simulink model "backbone"  (R2022b)
settings: Solver=FixedStepDiscrete  StartTime=0.0  StopTime=2  FixedStep=0.000001  RelTol=1e-3
undefined symbols (not defined in the file or in its folder): DiscIntNeverNeededParam, flux, Motor_flux, Motor_Ld_Indctances, Motor_Lq_Indctances, Motor_Pn, Motor_Rs, Pn, switch_electronic_feedworward, Switch_SubsysCtrl, SysCurrentMax, SysVoltage, Ts
libraries: powerlib_extras x11, simulink x4, mcbcontrolslib x4, slpidlib x3, spsPermanentMagnetSynchronousMachineLib x2, spsDCVoltageSourceLib x2, spsGroundLib x1, eePmsmCurrentController x1, spsThreePhaseVIMeasurementLib x1, spsTwoLevelConverterLib x1, spsUniversalBridgeLib x1, spspowerguiLib x1
(part 2 of 3)

== system backbone/Variant Subsystem/DTC_PMSM/PWM ==
  N : Inport
  Flux : Inport  Port=2
  Torque : Inport  Port=3
  Data Type Conversion : DataTypeConversion  OutDataTypeStr=boolean  SaturateOnIntegerOverflow=off  RndMeth=Floor
  Data Type Conversion1 : DataTypeConversion  OutDataTypeStr=boolean  SaturateOnIntegerOverflow=off  RndMeth=Floor
  Data Type Conversion2 : DataTypeConversion  OutDataTypeStr=boolean  SaturateOnIntegerOverflow=off  RndMeth=Floor
  Logical Operator3 : Logic  Operator=NOT  AllPortsSameDT=off  OutDataTypeStr=boolean
  Logical Operator4 : Logic  Operator=NOT  AllPortsSameDT=off  OutDataTypeStr=boolean
  Logical Operator5 : Logic  Operator=NOT  AllPortsSameDT=off  OutDataTypeStr=boolean
  Lookup Table : Lookup  InputValues=[1,2,3,4,5,6]  Table=[1,1,0,0,0,1]  SaturateOnIntegerOverflow=off
  Lookup Table1 : Lookup  InputValues=[1,2,3,4,5,6]  Table=[0,1,1,1,0,0]  SaturateOnIntegerOverflow=off
  Lookup Table2 : Lookup  InputValues=[1,2,3,4,5,6]  Table=[0,0,0,1,1,1]  SaturateOnIntegerOverflow=off
  Mux1 : Mux  Inputs=6
  PMSM_switch : MATLAB Function  TreatAsAtomicUnit=on
  pluse : Outport
  wires:
  Logical Operator3/1 -> Mux1/2
  Logical Operator4/1 -> Mux1/4
  Logical Operator5/1 -> Mux1/6
  Mux1/1 -> pluse/1
  PMSM_switch/1(Table) -> Lookup Table1/1, Lookup Table/1, Lookup Table2/1
  Lookup Table/1 -> Data Type Conversion/1
  Data Type Conversion/1 -> Mux1/1, Logical Operator3/1
  Lookup Table1/1 -> Data Type Conversion1/1
  Data Type Conversion1/1 -> Mux1/3, Logical Operator4/1
  Lookup Table2/1 -> Data Type Conversion2/1
  Data Type Conversion2/1 -> Mux1/5, Logical Operator5/1
  Flux/1 -> PMSM_switch/1(Flux)
  Torque/1 -> PMSM_switch/2(Torque)
  N/1 -> PMSM_switch/3(N)

== system backbone/Variant Subsystem/DTC_PMSM/Speed2 ==
  note: Pierre Giroux, Gilbert Sybille
      | Power System Simulation Laboratory
      | IREQ, Hydro-Quebc
  note: Discrete PID Controller
  Error : Inport  SampleTime=Ts
  Discrete-Time Integrator : DiscreteIntegrator  InitialCondition=Init  SampleTime=Ts  LimitOutput=on  UpperSaturationLimit=UpperLimit  LowerSaturationLimit=LowerLimit  ICPrevOutput=DiscIntNeverNeededParam  ICPrevScaledInput=DiscIntNeverNeededParam
  Kp1 : Gain  Gain=Ba  SaturateOnIntegerOverflow=on  SampleTime=Ts  OutDataTypeStr=Inherit: Same as input  ParamDataTypeStr=Inherit: Same as input
  Kp4 : Gain  Gain=Kpw  SaturateOnIntegerOverflow=on  SampleTime=Ts  OutDataTypeStr=Inherit: Same as input  ParamDataTypeStr=Inherit: Same as input
  Kp5 : Gain  Gain=Kiw  SaturateOnIntegerOverflow=on  SampleTime=Ts  OutDataTypeStr=Inherit: Same as input  ParamDataTypeStr=Inherit: Same as input
  Saturation2 : Saturate  UpperLimit=UpperLimit  LowerLimit=LowerLimit  SampleTime=Ts
  Sum6 : Sum  Inputs=++-  InputSameDT=on  SaturateOnIntegerOverflow=on  SampleTime=Ts  OutDataTypeStr=Inherit: Same as first input
  Zero-Order Hold : ZeroOrderHold  SampleTime=Ts
  Out : Outport  SampleTime=Ts  InitialOutput=0
  wires:
  Kp1/1 -> Sum6/3
  Sum6/1 -> Saturation2/1
  Kp5/1 -> Discrete-Time Integrator/1
  Kp4/1 -> Zero-Order Hold/1
  Discrete-Time Integrator/1 -> Sum6/2
  Saturation2/1 -> Out/1
  Zero-Order Hold/1 -> Sum6/1
  Error/1 -> Kp4/1, Kp5/1, Kp1/1

== system backbone/Variant Subsystem/DTC_PMSM/定子磁链和电磁转矩估计 ==
  note: 1) Add Subsystem or Model blocks as valid variant choices.
      | 2) You cannot connect blocks at this level. At simulation, connectivity is automatically
      | determined, based on the active variant and port name matching.
  Iα : Inport
  iβ : Inport  Port=2
  扩展卡尔曼滤波磁链估计 : Subsystem  VariantControl=DTC_Flux_Predict==2
  电压法估计磁链 : Subsystem  VariantControl=DTC_Flux_Predict==0
  N : Outport
  φ_est : Outport  Port=2
  Te_est : Outport  Port=3

== system backbone/Variant Subsystem/DTC_SVPWM_PMSM/速度pi1 ==
  note: Discrete PID Controller
  note: Pierre Giroux, Gilbert Sybille
      | Power System Simulation Laboratory
      | IREQ, Hydro-Quebc
  Error : Inport  SampleTime=Ts
  Discrete-Time Integrator : DiscreteIntegrator  InitialCondition=Init  SampleTime=Ts  LimitOutput=on  UpperSaturationLimit=UpperLimit  LowerSaturationLimit=LowerLimit  ICPrevOutput=DiscIntNeverNeededParam  ICPrevScaledInput=DiscIntNeverNeededParam
  Kp1 : Gain  Gain=Ba  SaturateOnIntegerOverflow=on  SampleTime=Ts  OutDataTypeStr=Inherit: Same as input  ParamDataTypeStr=Inherit: Same as input
  Kp4 : Gain  Gain=Kpw  SaturateOnIntegerOverflow=on  SampleTime=Ts  OutDataTypeStr=Inherit: Same as input  ParamDataTypeStr=Inherit: Same as input
  Kp5 : Gain  Gain=Kiw  SaturateOnIntegerOverflow=on  SampleTime=Ts  OutDataTypeStr=Inherit: Same as input  ParamDataTypeStr=Inherit: Same as input
  Saturation2 : Saturate  UpperLimit=UpperLimit  LowerLimit=LowerLimit  SampleTime=Ts
  Sum6 : Sum  Inputs=++-  InputSameDT=on  SaturateOnIntegerOverflow=on  SampleTime=Ts  OutDataTypeStr=Inherit: Same as first input
  Zero-Order Hold : ZeroOrderHold  SampleTime=Ts
  Out : Outport  SampleTime=Ts  InitialOutput=0
  wires:
  Error/1 -> Kp1/1, Kp5/1, Kp4/1
  Zero-Order Hold/1 -> Sum6/1
  Saturation2/1 -> Out/1
  Discrete-Time Integrator/1 -> Sum6/2
  Kp4/1 -> Zero-Order Hold/1
  Kp5/1 -> Discrete-Time Integrator/1
  Sum6/1 -> Saturation2/1
  Kp1/1 -> Sum6/3

== system backbone/Variant Subsystem/DTC_SVPWM_PMSM/速度pi2 ==
  note: Pierre Giroux, Gilbert Sybille
      | Power System Simulation Laboratory
      | IREQ, Hydro-Quebc
  note: Discrete PID Controller
  Error : Inport  SampleTime=Ts
  Discrete-Time Integrator : DiscreteIntegrator  InitialCondition=Init  SampleTime=Ts  LimitOutput=on  UpperSaturationLimit=UpperLimit  LowerSaturationLimit=LowerLimit  ICPrevOutput=DiscIntNeverNeededParam  ICPrevScaledInput=DiscIntNeverNeededParam
  Kp1 : Gain  Gain=Ba  SaturateOnIntegerOverflow=on  SampleTime=Ts  OutDataTypeStr=Inherit: Same as input  ParamDataTypeStr=Inherit: Same as input
  Kp4 : Gain  Gain=Kpw  SaturateOnIntegerOverflow=on  SampleTime=Ts  OutDataTypeStr=Inherit: Same as input  ParamDataTypeStr=Inherit: Same as input
  Kp5 : Gain  Gain=Kiw  SaturateOnIntegerOverflow=on  SampleTime=Ts  OutDataTypeStr=Inherit: Same as input  ParamDataTypeStr=Inherit: Same as input
  Saturation2 : Saturate  UpperLimit=UpperLimit  LowerLimit=LowerLimit  SampleTime=Ts
  Sum6 : Sum  Inputs=++-  InputSameDT=on  SaturateOnIntegerOverflow=on  SampleTime=Ts  OutDataTypeStr=Inherit: Same as first input
  Zero-Order Hold : ZeroOrderHold  SampleTime=Ts
  Out : Outport  SampleTime=Ts  InitialOutput=0
  wires:
  Kp1/1 -> Sum6/3
  Sum6/1 -> Saturation2/1
  Kp5/1 -> Discrete-Time Integrator/1
  Kp4/1 -> Zero-Order Hold/1
  Discrete-Time Integrator/1 -> Sum6/2
  Saturation2/1 -> Out/1
  Zero-Order Hold/1 -> Sum6/1
  Error/1 -> Kp4/1, Kp5/1, Kp1/1

== system backbone/Variant Subsystem/MPTA_MPTV_PMSM/Back Electromotive Force ==
  note: (We*Lq*iq)
  note: We*flux
  note: (We*Ld*id)
  we : Inport
  iq : Inport  Port=2
  id : Inport  Port=3
  Constant : Constant  Value=0
  Constant1 : Constant  Value=switch_electronic_feedworward
  Gain : Gain  Gain=Motor_Ld_Indctances
  Gain1 : Gain  Gain=Motor_flux
  Gain2 : Gain  Gain=Motor_Lq_Indctances
  Product : Product
  Product1 : Product
  Sum : Sum
  Switch : Switch  Criteria=u2 > Threshold  SaturateOnIntegerOverflow=off  InputSameDT=off
  E_d : Outport
  E_q : Outport  Port=2
  wires:
  Switch/1 -> Gain1/1, Gain/1, Gain2/1
  Product1/1 -> E_d/1
  Gain1/1 -> Sum/1
  Sum/1 -> E_q/1
  Product/1 -> Sum/2
  Constant1/1 -> Switch/2
  id/1 -> Product/2
  iq/1 -> Product1/2
  Gain2/1 -> Product1/1
  Gain/1 -> Product/1
  we/1 -> Switch/1
  Constant/1 -> Switch/3

== system backbone/Variant Subsystem/MPTA_MPTV_PMSM/MPTA_弱磁 ==
  note: 1) Add Subsystem or Model blocks as valid variant choices.
      | 2) You cannot connect blocks at this level. At simulation, connectivity is automatically
      | determined, based on the active variant and port name matching.
  input : Inport
  "MPTA_MPTV_Base_IMax " : Subsystem  VariantControl=true
  MPTA_MPTV_Base_Te : Subsystem  VariantControl=false
  id_ref : Outport
  iq_ref : Outport  Port=2

== system backbone/Variant Subsystem/SMC_OR_PID/Back Electromotive Force ==
  note: (We*Ld*id)
  note: (We*flux)
  note: (We*Lq*iq)
  we : Inport
  iq : Inport  Port=2
  id : Inport  Port=3
  Constant : Constant  Value=0
  Constant1 : Constant  Value=switch_electronic_feedworward
  Gain : Gain  Gain=Motor_Ld_Indctances
  Gain1 : Gain  Gain=Motor_flux
  Gain2 : Gain  Gain=Motor_Lq_Indctances
  Product : Product
  Product1 : Product
  Sum : Sum
  Switch : Switch  Criteria=u2 > Threshold  SaturateOnIntegerOverflow=off  InputSameDT=off
  E_d : Outport
  E_q : Outport  Port=2
  wires:
  Gain/1 -> Product/1
  Gain2/1 -> Product1/1
  iq/1 -> Product1/2
  id/1 -> Product/2
  Constant1/1 -> Switch/2
  Product/1 -> Sum/2
  Sum/1 -> E_q/1
  Gain1/1 -> Sum/1
  Product1/1 -> E_d/1
  Switch/1 -> Gain2/1, Gain/1, Gain1/1
  Constant/1 -> Switch/3
  we/1 -> Switch/1

== system backbone/Variant Subsystem/SMC_OR_PID/Variant Subsystem ==
  note: 1) Add Subsystem or Model blocks as valid variant choices.
      | 2) You cannot connect blocks at this level. At simulation, connectivity is automatically
      | determined, based on the active variant and port name matching.
  In1 : Inport
  PID : Subsystem  VariantControl=true
  SMC : Subsystem  VariantControl=false
  Te* : Outport

== system backbone/Variant Subsystem/SMC_OR_PID/Variant Subsystem1 ==
  note: 1) Add Subsystem or Model blocks as valid variant choices.
      | 2) You cannot connect blocks at this level. At simulation, connectivity is automatically
      | determined, based on the active variant and port name matching.
  we : Inport
  Te* : Inport  Port=2
  LD=LQ/id=0 : Subsystem  VariantControl=MPTA_SubSysCtrl==0
  MPTA_Process : Subsystem  VariantControl=MPTA_SubSysCtrl==1
  id_ref : Outport
  iq_ref : Outport  Port=2

== system backbone/Variant Subsystem/SMC_OR_PID/Variant Subsystem2 ==
  note: 1) Add Subsystem or Model blocks as valid variant choices.
      | 2) You cannot connect blocks at this level. At simulation, connectivity is automatically
      | determined, based on the active variant and port name matching.
  ialpha : Inport
  ibeta : Inport  Port=2
  ualpha : Inport  Port=3
  ubeta : Inport  Port=4
  Ts : Inport  Port=5
  Ls : Inport  Port=6
  Rs : Inport  Port=7
  flux : Inport  Port=8
  EKF_dq : Subsystem  VariantControl=(Motor_Observer==2)&&(Motor_Ld_Indctances==Motor_Lq_Indctances)
  EKF_αβ : Subsystem  VariantControl=Motor_Observer==0
  Luenberger : Subsystem  VariantControl=Motor_Observer==1
  Model : ModelReference  VariantControl=Choice
  SMO : Subsystem  VariantControl=Motor_Observer==3
  theta : Outport
  we : Outport  Port=2

== system backbone/输出模拟子系统/磁链模拟/Variant Subsystem ==
  note: 1) Add Subsystem or Model blocks as valid variant choices.
      | 2) You cannot connect blocks at this level. At simulation, connectivity is automatically
      | determined, based on the active variant and port name matching.
  In1 : Inport
  Subsystem : Subsystem  VariantControl=true
  Subsystem1 : Subsystem  VariantControl=false
  Out1 : Outport

== system backbone/输出模拟子系统/磁链模拟/clark变换 ==
  note: 基于KCL定律消除Ic 减少一路电流检测，简化clark变换计算过程
  i_a : Inport
  i_b : Inport  Port=2
  i_c : Inport  Port=3
  " 1" : Fcn  Expr=u(1)*(3/2)
  " 1" : Fcn  Expr=u(1)*(sqrt(3)/2)+u(2)*(sqrt(3))
  Mux7 : Mux  Inputs=3
  Alpha : Outport
  Beta : Outport  Port=2
  wires:
  " 1"/1 -> Alpha/1
  " 1"/1 -> Beta/1
  Mux7/1 -> " 1"/1, " 1"/1
  i_a/1 -> Mux7/1
  i_b/1 -> Mux7/2
  i_c/1 -> Mux7/3

== system backbone/输出模拟子系统/磁链模拟/park变换 ==
  Alpha : Inport
  Beta : Inport  Port=2
  We : Inport  Port=3
  " 1" : Fcn  Expr=u(1)*cos(u(3))+u(2)*sin(u(3))
  " 1" : Scope  NumInputPorts=2
  " 1" : Fcn  Expr=-u(1)*sin(u(3))+u(2)*cos(u(3))
  Mux8 : Mux  Inputs=3
  D : Outport
  Q : Outport  Port=2
  wires:
  Alpha/1 -> Mux8/1
  Beta/1 -> Mux8/2
  Mux8/1 -> " 1"/1, " 1"/1
  We/1 -> Mux8/3
  " 1"/1 -> " 1"/1, D/1
  " 1"/1 -> " 1"/2, Q/1

== system backbone/Variant Subsystem/DTC_PMSM/定子磁链和电磁转矩估计/扩展卡尔曼滤波磁链估计 ==
  Iα : Inport
  iβ : Inport  Port=2
  φ_est : Outport
  Te_est : Outport  Port=2
  N : Outport  Port=3

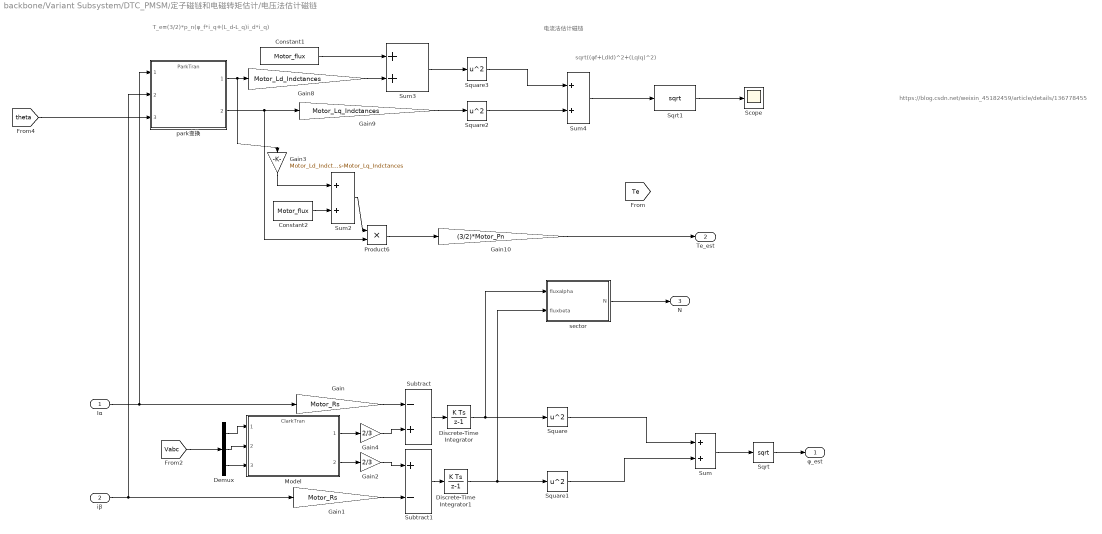
== system backbone/Variant Subsystem/DTC_PMSM/定子磁链和电磁转矩估计/电压法估计磁链 ==
  note: T_e=(3/2)*p_n(φ_f*i_q+(L_d-L_q)i_d*i_q)
  note: 电流法估计磁链
  note: sqrt((φf+LdId)^2+(LqIq)^2)
  note: https://blog.csdn.net/weixin_45182459/article/details/136778455
  Iα : Inport
  iβ : Inport  Port=2
  Constant1 : Constant  Value=Motor_flux
  Constant2 : Constant  Value=Motor_flux
  Demux : Demux  Outputs=3
  Discrete-Time Integrator : DiscreteIntegrator  SampleTime=-1  ICPrevOutput=DiscIntNeverNeededParam  ICPrevScaledInput=DiscIntNeverNeededParam
  Discrete-Time Integrator1 : DiscreteIntegrator  SampleTime=-1  ICPrevOutput=DiscIntNeverNeededParam  ICPrevScaledInput=DiscIntNeverNeededParam
  Gain : Gain  Gain=Motor_Rs
  Gain1 : Gain  Gain=Motor_Rs
  Gain10 : Gain  Gain=(3/2)*Motor_Pn
  Gain2 : Gain  Gain=2/3
  Gain3 : Gain  Gain=Motor_Ld_Indctances-Motor_Lq_Indctances
  Gain4 : Gain  Gain=2/3
  Gain8 : Gain  Gain=Motor_Ld_Indctances
  Gain9 : Gain  Gain=Motor_Lq_Indctances
  Model : ModelReference  ModelNameDialog=ClarkTran.slx  SimulationMode=Normal  ModelReferenceVersion=1.13
  Product6 : Product
  Scope : Scope
  Sqrt : Sqrt
  Sqrt1 : Sqrt
  Square{,1..3} (4 alike) : Math  Operator=square
  Subtract : Sum  Inputs=-+
  Subtract1 : Sum  Inputs=+-
  Sum{,2..4} (4 alike) : Sum
  park变换 : ModelReference  ModelNameDialog=ParkTran.slx  SimulationMode=Normal  ModelReferenceVersion=1.9
  sector : MATLAB Function  TreatAsAtomicUnit=on
  φ_est : Outport
  Te_est : Outport  Port=2
  N : Outport  Port=3
  wires:
  [Vabc] -> Demux/1
  Demux/1 -> Model/1
  Demux/2 -> Model/2
  Demux/3 -> Model/3
  Gain/1 -> Subtract/1
  Gain1/1 -> Subtract1/2
  Subtract/1 -> Discrete-Time Integrator/1
  Subtract1/1 -> Discrete-Time Integrator1/1
  Square/1 -> Sum/1
  Square1/1 -> Sum/2
  Sum/1 -> Sqrt/1
  Sqrt/1 -> φ_est/1
  sector/1(N) -> N/1
  Gain2/1 -> Subtract1/1
  Model/2 -> Gain2/1
  Gain4/1 -> Subtract/2
  Model/1 -> Gain4/1
  Iα/1 -> park变换/1, Gain/1
  Discrete-Time Integrator/1 -> sector/1(fluxalpha), Square/1
  Discrete-Time Integrator1/1 -> sector/2(fluxbeta), Square1/1
  Constant2/1 -> Sum2/2
  park变换/2 -> Product6/2, Gain9/1
  park变换/1 -> Gain3/1, Gain8/1
  Gain8/1 -> Sum3/2
  Constant1/1 -> Sum3/1
  Product6/1 -> Gain10/1
  Sum2/1 -> Product6/1
  Gain3/1 -> Sum2/1
  Square3/1 -> Sum4/1
  Gain9/1 -> Square2/1
  Square2/1 -> Sum4/2
  Sum3/1 -> Square3/1
  Sum4/1 -> Sqrt1/1
  [theta] -> park变换/3
  Sqrt1/1 -> Scope/1
  iβ/1 -> park变换/2, Gain1/1
  Gain10/1 -> Te_est/1

== system backbone/Variant Subsystem/MPTA_MPTV_PMSM/MPTA_弱磁/MPTA_MPTV_Base_IMax  ==
  note: [57.6177 -57.6177]
  note: [50*sqrt(2) -50*sqrt(2)]
  note: https://blog.csdn.net/weixin_44312889/article/details/124467496
  note: https://blog.csdn.net/weixin_44312889/article/details/124467496?ops_request_misc=%257B%2522request%255Fid%2522%253A%2522171975641716800215087501%2522%252C%2522scm%2522%253A%252220140713.130102334.pc%255Fblog.%2522%257D&request_id=171975641716800215087501&biz_id=0&utm_medium=distribute.pc_search_result.none-task-blog-2~blog~first_rank_ecpm_v1~rank_v31_ecpm-23-124467496-null-null.nonecase&utm_term=%20%E5%BC%B1%E7%A3%81%E6%8E%A7%E5%88%B6&spm=1018.2226.3001.4450
  note: https://www.bilibili.com/video/BV1iZ421v75g/?spm_id_from=333.337.search-card.all.click&vd_source=a44fa1878c4911e289ac9693c05baa9b
  note: 此处PID 对应着转速与iq的关系
  input : Inport
  Clock : Clock
  Delay : Delay  DelayLength=1
  LdLqPnFluxRs : Constant  Value=[Motor_Ld_Indctances Motor_Lq_Indctances Motor_Pn Motor_flux Motor_Rs]
  MPTA_MPTV_Imax : MATLAB Function  TreatAsAtomicUnit=on
  MPTA_MPTV_Imax1 : MATLAB Function  Commented=on  TreatAsAtomicUnit=on
  Scope : Scope
  Speed : Subsystem  AncestorBlock=|  DialogController=POWERSYS.PowerSysDialog  mask(Discrete PI Controller){Kpw=0.075, Kiw=0.4, Ba=0, Par_Limits=[57.7 -5], Init=0, Ts=1e-3}
      | powerlib_extras/Discrete 
      | Control Blocks/Discrete
      | PI Controller
      mask prompts: Kpw "Proportional gain (Kp):"; Kiw "Integral gain (Ki):"; Ba "feedback gain (Ba)"; Par_Limits "Output limits: [ Upper   Lower ]"; Init "Output initial value:"; Ts "Sample time:"
      mask help: This block implements a discrete PI controller.
      mask init:
      | UpperLimit=Par_Limits(1);
      | LowerLimit=Par_Limits(2);
      | power_initmask();
      settings: LibrarySourceBlock=|
      | powerlib_extras/Discrete
      | Control Blocks/Discrete
      | PI Controller
      mask Help: This block is part of a subset of blocks in the Extras library that does not have documentation associated with it, other than the block mask description.
      mask Display: disp('PI');
  UI : Constant  Value=[SysVoltage SysCurrentMax]
  iq_ref : Outport
  id_ref : Outport  Port=2
  wires:
  UI/1 -> MPTA_MPTV_Imax/2(UI)
  Delay/1 -> MPTA_MPTV_Imax/6(last_state)
  [we] -> MPTA_MPTV_Imax/5(we)
  Clock/1 -> MPTA_MPTV_Imax/4(clock)
  MPTA_MPTV_Imax/3(state) -> Delay/1
  LdLqPnFluxRs/1 -> MPTA_MPTV_Imax/3(LdLqPnFluxRs)
  input/1 -> Speed/1(Error)
  Speed/1(Out) -> MPTA_MPTV_Imax/1(iqPIDref)
  MPTA_MPTV_Imax/6(Zone) -> Scope/1
  MPTA_MPTV_Imax/2(iqref) -> iq_ref/1
  MPTA_MPTV_Imax/1(idref) -> id_ref/1

== system backbone/Variant Subsystem/MPTA_MPTV_PMSM/MPTA_弱磁/MPTA_MPTV_Base_Te ==
  note: https://blog.csdn.net/qq_54203407/article/details/133353778
  note: https://blog.csdn.net/qq_54203407/article/details/133353778?ops_request_misc=%257B%2522request%255Fid%2522%253A%2522171984152416800225547611%2522%252C%2522scm%2522%253A%252220140713.130102334..%2522%257D&request_id=171984152416800225547611&biz_id=0&utm_medium=distribute.pc_search_result.none-task-blog-2~blog~sobaiduend~default-2-133353778-null-null.nonecase&utm_term=mpta&spm=1018.2226.3001.4450
  note: 此处PID 对应着转速和转矩的关系
  input : Inport
  LdLqPnFluxRs : Constant  Value=[Motor_Ld_Indctances Motor_Lq_Indctances Motor_Pn Motor_flux Motor_Rs]
  MPTA_MPTV_Imax : MATLAB Function  TreatAsAtomicUnit=on
  UI : Constant  Value=[SysVoltage SysCurrentMax]
  Variant Subsystem : Subsystem  Variant=on
  iq_ref : Outport
  id_ref : Outport  Port=2
  wires:
  LdLqPnFluxRs/1 -> MPTA_MPTV_Imax/4(LdLqPnFluxRs)
  input/1 -> Variant Subsystem/1(In1)
  Variant Subsystem/1(Te*) -> MPTA_MPTV_Imax/2(iqref_raw)
  UI/1 -> MPTA_MPTV_Imax/3(UI)
  [we] -> MPTA_MPTV_Imax/5(we)
  MPTA_MPTV_Imax/1(idref) -> id_ref/1
  MPTA_MPTV_Imax/2(iqref) -> iq_ref/1

== system backbone/Variant Subsystem/SMC_OR_PID/Variant Subsystem/PID ==
  In1 : Inport
  Speed1 : Subsystem  AncestorBlock=|  DialogController=POWERSYS.PowerSysDialog  mask(Discrete PI Controller){Kpw=0.073, Kiw=0.12, Ba=0, Par_Limits=[50*sqrt(2) -50*sqrt(2)], Init=0, Ts=1e-6}
      | powerlib_extras/Discrete 
      | Control Blocks/Discrete
      | PI Controller
      mask prompts: Kpw "Proportional gain (Kp):"; Kiw "Integral gain (Ki):"; Ba "feedback gain (Ba)"; Par_Limits "Output limits: [ Upper   Lower ]"; Init "Output initial value:"; Ts "Sample time:"
      mask help: This block implements a discrete PI controller.
      mask init:
      | UpperLimit=Par_Limits(1);
      | LowerLimit=Par_Limits(2);
      | power_initmask();
      settings: LibrarySourceBlock=|
      | powerlib_extras/Discrete
      | Control Blocks/Discrete
      | PI Controller
      mask Help: This block is part of a subset of blocks in the Extras library that does not have documentation associated with it, other than the block mask description.
      mask Display: disp('PI');
  Speed2 : Subsystem  Commented=on  AncestorBlock=|  DialogController=POWERSYS.PowerSysDialog  mask(Discrete PI Controller){Kpw=0.14, Kiw=0.14*50, Ba=0, Par_Limits=[800 -800], Init=0, Ts=Ts}
      | powerlib_extras/Discrete 
      | Control Blocks/Discrete
      | PI Controller
      mask prompts: Kpw "Proportional gain (Kp):"; Kiw "Integral gain (Ki):"; Ba "feedback gain (Ba)"; Par_Limits "Output limits: [ Upper   Lower ]"; Init "Output initial value:"; Ts "Sample time:"
      mask help: This block implements a discrete PI controller.
      mask init:
      | UpperLimit=Par_Limits(1);
      | LowerLimit=Par_Limits(2);
      | power_initmask();
      settings: LibrarySourceBlock=|
      | powerlib_extras/Discrete
      | Control Blocks/Discrete
      | PI Controller
      mask Help: This block is part of a subset of blocks in the Extras library that does not have documentation associated with it, other than the block mask description.
      mask Display: disp('PI');
  Te* : Outport
  wires:
  In1/1 -> Speed1/1(Error)
  Speed1/1(Out) -> Te*/1

== system backbone/Variant Subsystem/SMC_OR_PID/Variant Subsystem/SMC ==
  In1 : Inport
  Speed4 : Subsystem  AncestorBlock=|  DialogController=POWERSYS.PowerSysDialog  mask(Discrete PI Controller){C=60, Mu=200, q=300, Par_Limits=[1000 -1000], Init=0, Ts=0.000001}
      | powerlib_extras/Discrete 
      | Control Blocks/Discrete
      | PI Controller
      mask prompts: C "Gain (c):"; Mu "Gain (Mu):"; q "Gain (q)"; Par_Limits "Output limits: [ Upper   Lower ]"; Init "Output initial value:"; Ts "Sample time:"
      mask help: This block implements a discrete PI controller.
      mask init:
      | UpperLimit=Par_Limits(1);
      | LowerLimit=Par_Limits(2);
      | power_initmask();
      settings: LibrarySourceBlock=|
      | powerlib_extras/Discrete
      | Control Blocks/Discrete
      | PI Controller
      mask Help: This block is part of a subset of blocks in the Extras library that does not have documentation associated with it, other than the block mask description.
      mask Display: disp('SMC');
  Te* : Outport
  wires:
  In1/1 -> Speed4/1(Error)
  Speed4/1(Out) -> Te*/1

== system backbone/Variant Subsystem/SMC_OR_PID/Variant Subsystem1/LD=LQ//id=0 ==
  Te* : Inport
  we : Inport  Port=2
  Constant : Constant  Value=0
  id_ref : Outport
  iq_ref : Outport  Port=2
  wires:
  Constant/1 -> id_ref/1
  Te*/1 -> iq_ref/1

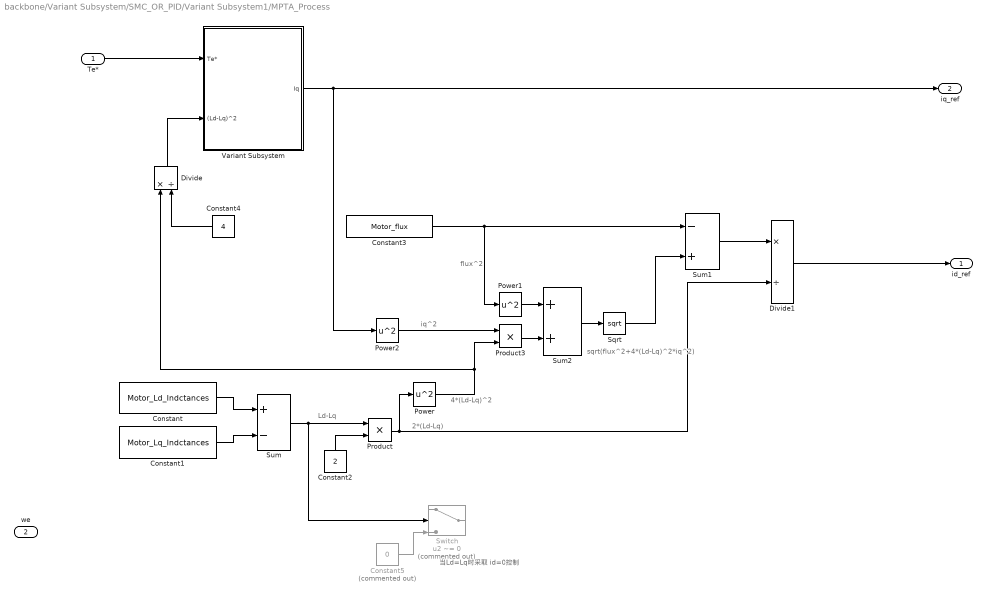
== system backbone/Variant Subsystem/SMC_OR_PID/Variant Subsystem1/MPTA_Process ==
  note: 当Ld=Lq时采取 id=0控制
  note: 4*(Ld-Lq)^2
  note: 2*(Ld-Lq)
  note: Ld-Lq
  note: iq^2
  note: flux^2
  note: sqrt(flux^2+4*(Ld-Lq)^2*iq^2)
  Te* : Inport
  we : Inport  Port=2
  Constant : Constant  Value=Motor_Ld_Indctances
  Constant1 : Constant  Value=Motor_Lq_Indctances
  Constant2 : Constant  Value=2
  Constant3 : Constant  Value=Motor_flux
  Constant4 : Constant  Value=4
  Constant5 : Constant  Commented=on  Value=0
  Divide : Product  Inputs=*/
  Divide1 : Product  Inputs=*/
  Power : Math  Operator=square
  Power1 : Math  Operator=square
  Power2 : Math  Operator=square
  Product : Product
  Product3 : Product
  Sqrt : Sqrt
  Sum : Sum  Inputs=+-
  Sum1 : Sum  Inputs=-+
  Sum2 : Sum
  Switch : Switch  Commented=on  Criteria=u2 ~= 0  SaturateOnIntegerOverflow=off  InputSameDT=off
  Variant Subsystem : Subsystem  Variant=on
  id_ref : Outport
  iq_ref : Outport  Port=2
  wires:
  Constant1/1 -> Sum/2
  Sum1/1 -> Divide1/1
  Power1/1 -> Sum2/1
  Power2/1 -> Product3/1
  Variant Subsystem/1(Iq) -> iq_ref/1, Power2/1
  Power/1 -> Divide/1, Product3/2
  Te*/1 -> Variant Subsystem/1(Te*)
  Sum2/1 -> Sqrt/1
  Sqrt/1 -> Sum1/2
  Constant4/1 -> Divide/2
  Product/1 -> Divide1/2, Power/1
  Divide/1 -> Variant Subsystem/2((Ld-Lq)^2)
  Constant2/1 -> Product/2
  Constant/1 -> Sum/1
  Product3/1 -> Sum2/2
  Constant3/1 -> Sum1/1, Power1/1
  Sum/1 -> Switch/2, Product/1
  Constant5/1 -> Switch/3
  Divide1/1 -> id_ref/1

== system backbone/Variant Subsystem/SMC_OR_PID/Variant Subsystem2/EKF_dq ==
  ialpha : Inport
  theta : Outport

== system backbone/Variant Subsystem/SMC_OR_PID/Variant Subsystem2/EKF_αβ ==
  ialpha : Inport
  ibeta : Inport  Port=2
  ualpha : Inport  Port=3
  ubeta : Inport  Port=4
  Ts : Inport  Port=5
  Ls : Inport  Port=6
  Rs : Inport  Port=7
  flux : Inport  Port=8
  Delay : Delay  DelayLength=1
  Delay1 : Delay  DelayLength=1
  MATLAB Function : MATLAB Function  TreatAsAtomicUnit=on
  theta : Outport
  we : Outport  Port=2
  wires:
  ialpha/1 -> MATLAB Function/1(ialpha)
  ibeta/1 -> MATLAB Function/2(ibeta)
  ualpha/1 -> MATLAB Function/3(ualpha)
  ubeta/1 -> MATLAB Function/4(ubeta)
  Ts/1 -> MATLAB Function/5(Ts)
  Ls/1 -> MATLAB Function/6(Ls)
  Rs/1 -> MATLAB Function/7(Rs)
  flux/1 -> MATLAB Function/8(flux)
  MATLAB Function/1(theta) -> Delay/1
  MATLAB Function/2(we) -> Delay1/1
  Delay/1 -> theta/1
  Delay1/1 -> we/1

== system backbone/Variant Subsystem/SMC_OR_PID/Variant Subsystem2/Luenberger ==
  ialpha : Inport
  theta : Outport

== system backbone/Variant Subsystem/SMC_OR_PID/Variant Subsystem2/SMO ==
  ialpha : Inport
  theta : Outport

== system backbone/输出模拟子系统/磁链模拟/Variant Subsystem/Subsystem ==
  In1 : Inport
  Out1 : Outport

== system backbone/输出模拟子系统/磁链模拟/Variant Subsystem/Subsystem1 ==
  In1 : Inport
  Out1 : Outport

== system backbone/Variant Subsystem/MPTA_MPTV_PMSM/MPTA_弱磁/MPTA_MPTV_Base_IMax /Speed ==
  note: Pierre Giroux, Gilbert Sybille
      | Power System Simulation Laboratory
      | IREQ, Hydro-Quebc
  note: Discrete PID Controller
  Error : Inport  SampleTime=Ts
  Discrete-Time Integrator : DiscreteIntegrator  InitialCondition=Init  SampleTime=Ts  LimitOutput=on  UpperSaturationLimit=UpperLimit  LowerSaturationLimit=LowerLimit  ICPrevOutput=DiscIntNeverNeededParam  ICPrevScaledInput=DiscIntNeverNeededParam
  Kp1 : Gain  Gain=Ba  SaturateOnIntegerOverflow=on  SampleTime=Ts  OutDataTypeStr=Inherit: Same as input  ParamDataTypeStr=Inherit: Same as input
  Kp4 : Gain  Gain=Kpw  SaturateOnIntegerOverflow=on  SampleTime=Ts  OutDataTypeStr=Inherit: Same as input  ParamDataTypeStr=Inherit: Same as input
  Kp5 : Gain  Gain=Kiw  SaturateOnIntegerOverflow=on  SampleTime=Ts  OutDataTypeStr=Inherit: Same as input  ParamDataTypeStr=Inherit: Same as input
  Saturation2 : Saturate  UpperLimit=UpperLimit  LowerLimit=LowerLimit  SampleTime=Ts
  Sum6 : Sum  Inputs=++-  InputSameDT=on  SaturateOnIntegerOverflow=on  SampleTime=Ts  OutDataTypeStr=Inherit: Same as first input
  Zero-Order Hold : ZeroOrderHold  SampleTime=Ts
  Out : Outport  SampleTime=Ts  InitialOutput=0
  wires:
  Kp1/1 -> Sum6/3
  Sum6/1 -> Saturation2/1
  Kp5/1 -> Discrete-Time Integrator/1
  Kp4/1 -> Zero-Order Hold/1
  Discrete-Time Integrator/1 -> Sum6/2
  Saturation2/1 -> Out/1
  Zero-Order Hold/1 -> Sum6/1
  Error/1 -> Kp4/1, Kp5/1, Kp1/1

== system backbone/Variant Subsystem/MPTA_MPTV_PMSM/MPTA_弱磁/MPTA_MPTV_Base_Te/Variant Subsystem ==
  note: 1) Add Subsystem or Model blocks as valid variant choices.
      | 2) You cannot connect blocks at this level. At simulation, connectivity is automatically
      | determined, based on the active variant and port name matching.
  In1 : Inport
  PID : Subsystem  VariantControl=true
  SMC : Subsystem  VariantControl=false
  Te* : Outport

== system backbone/Variant Subsystem/SMC_OR_PID/Variant Subsystem/PID/Speed1 ==
  note: Pierre Giroux, Gilbert Sybille
      | Power System Simulation Laboratory
      | IREQ, Hydro-Quebc
  note: Discrete PID Controller
  Error : Inport  SampleTime=Ts
  Discrete-Time Integrator : DiscreteIntegrator  InitialCondition=Init  SampleTime=Ts  LimitOutput=on  UpperSaturationLimit=UpperLimit  LowerSaturationLimit=LowerLimit  ICPrevOutput=DiscIntNeverNeededParam  ICPrevScaledInput=DiscIntNeverNeededParam
  Kp1 : Gain  Gain=Ba  SaturateOnIntegerOverflow=on  SampleTime=Ts  OutDataTypeStr=Inherit: Same as input  ParamDataTypeStr=Inherit: Same as input
  Kp4 : Gain  Gain=Kpw  SaturateOnIntegerOverflow=on  SampleTime=Ts  OutDataTypeStr=Inherit: Same as input  ParamDataTypeStr=Inherit: Same as input
  Kp5 : Gain  Gain=Kiw  SaturateOnIntegerOverflow=on  SampleTime=Ts  OutDataTypeStr=Inherit: Same as input  ParamDataTypeStr=Inherit: Same as input
  Saturation2 : Saturate  UpperLimit=UpperLimit  LowerLimit=LowerLimit  SampleTime=Ts
  Sum6 : Sum  Inputs=++-  InputSameDT=on  SaturateOnIntegerOverflow=on  SampleTime=Ts  OutDataTypeStr=Inherit: Same as first input
  Zero-Order Hold : ZeroOrderHold  SampleTime=Ts
  Out : Outport  SampleTime=Ts  InitialOutput=0
  wires:
  Kp1/1 -> Sum6/3
  Sum6/1 -> Saturation2/1
  Kp5/1 -> Discrete-Time Integrator/1
  Kp4/1 -> Zero-Order Hold/1
  Discrete-Time Integrator/1 -> Sum6/2
  Saturation2/1 -> Out/1
  Zero-Order Hold/1 -> Sum6/1
  Error/1 -> Kp4/1, Kp5/1, Kp1/1

== system backbone/Variant Subsystem/SMC_OR_PID/Variant Subsystem/PID/Speed2 ==
  note: Pierre Giroux, Gilbert Sybille
      | Power System Simulation Laboratory
      | IREQ, Hydro-Quebc
  note: Discrete PID Controller
  Error : Inport  SampleTime=Ts
  Discrete-Time Integrator : DiscreteIntegrator  InitialCondition=Init  SampleTime=Ts  LimitOutput=on  UpperSaturationLimit=UpperLimit  LowerSaturationLimit=LowerLimit  ICPrevOutput=DiscIntNeverNeededParam  ICPrevScaledInput=DiscIntNeverNeededParam
  Kp1 : Gain  Gain=Ba  SaturateOnIntegerOverflow=on  SampleTime=Ts  OutDataTypeStr=Inherit: Same as input  ParamDataTypeStr=Inherit: Same as input
  Kp4 : Gain  Gain=Kpw  SaturateOnIntegerOverflow=on  SampleTime=Ts  OutDataTypeStr=Inherit: Same as input  ParamDataTypeStr=Inherit: Same as input
  Kp5 : Gain  Gain=Kiw  SaturateOnIntegerOverflow=on  SampleTime=Ts  OutDataTypeStr=Inherit: Same as input  ParamDataTypeStr=Inherit: Same as input
  Saturation2 : Saturate  UpperLimit=UpperLimit  LowerLimit=LowerLimit  SampleTime=Ts
  Sum6 : Sum  Inputs=++-  InputSameDT=on  SaturateOnIntegerOverflow=on  SampleTime=Ts  OutDataTypeStr=Inherit: Same as first input
  Zero-Order Hold : ZeroOrderHold  SampleTime=Ts
  Out : Outport  SampleTime=Ts  InitialOutput=0
  wires:
  Kp1/1 -> Sum6/3
  Sum6/1 -> Saturation2/1
  Kp5/1 -> Discrete-Time Integrator/1
  Kp4/1 -> Zero-Order Hold/1
  Discrete-Time Integrator/1 -> Sum6/2
  Saturation2/1 -> Out/1
  Zero-Order Hold/1 -> Sum6/1
  Error/1 -> Kp4/1, Kp5/1, Kp1/1

== system backbone/Variant Subsystem/SMC_OR_PID/Variant Subsystem/SMC/Speed4 ==
  Error : Inport  SampleTime=Ts
  1/D : Gain  Gain=1/(1.5*Pn*flux/0.003)  SaturateOnIntegerOverflow=on  SampleTime=Ts  OutDataTypeStr=Inherit: Same as input  ParamDataTypeStr=Inherit: Same as input
  Discrete Derivative : simulink/Discrete/Discrete Derivative  gainval=1.0  ICPrevScaledInput=0.0  OutMin=[]  OutMax=[]  OutDataType=fixdt(1, 16)  OutScaling=2^-10  DoSatur=off
  Discrete-Time Integrator : DiscreteIntegrator  InitialCondition=0.001  SampleTime=Ts  ICPrevOutput=DiscIntNeverNeededParam  ICPrevScaledInput=DiscIntNeverNeededParam
  Kp1 : Gain  Gain=q  SaturateOnIntegerOverflow=on  SampleTime=Ts  OutDataTypeStr=Inherit: Same as input  ParamDataTypeStr=Inherit: Same as input
  Kp2 : Gain  Gain=Mu  SaturateOnIntegerOverflow=on  SampleTime=Ts  OutDataTypeStr=Inherit: Same as input  ParamDataTypeStr=Inherit: Same as input
  Kp3 : Gain  Gain=C  SaturateOnIntegerOverflow=on  SampleTime=Ts  OutDataTypeStr=Inherit: Same as input  ParamDataTypeStr=Inherit: Same as input
  Kp4 : Gain  Gain=C  SaturateOnIntegerOverflow=on  SampleTime=Ts  OutDataTypeStr=Inherit: Same as input  ParamDataTypeStr=Inherit: Same as input
  Nr->wm : Gain  Gain=pi/30  SaturateOnIntegerOverflow=on  SampleTime=Ts  OutDataTypeStr=Inherit: Same as input  ParamDataTypeStr=Inherit: Same as input
  Saturation2 : Saturate  UpperLimit=UpperLimit  LowerLimit=LowerLimit  SampleTime=Ts
  Sign : Signum
  Sum1 : Sum  InputSameDT=on  SaturateOnIntegerOverflow=on  SampleTime=Ts  OutDataTypeStr=Inherit: Same as first input
  Sum2 : Sum  Inputs=++-  InputSameDT=on  SaturateOnIntegerOverflow=on  SampleTime=Ts  OutDataTypeStr=Inherit: Same as first input
  Out : Outport  SampleTime=Ts  InitialOutput=0
  wires:
  Kp4/1 -> Sum1/1
  Saturation2/1 -> Out/1
  Discrete Derivative/1 -> Kp3/1, Sum1/2
  Sum2/1 -> Discrete-Time Integrator/1
  Error/1 -> Nr->wm/1
  Kp1/1 -> Sum2/1
  Sign/1 -> Kp2/1
  Sum1/1 -> Sign/1, Kp1/1
  Kp2/1 -> Sum2/2
  Kp3/1 -> Sum2/3
  1/D/1 -> Saturation2/1
  Discrete-Time Integrator/1 -> 1/D/1
  Nr->wm/1 -> Discrete Derivative/1, Kp4/1

== system backbone/Variant Subsystem/SMC_OR_PID/Variant Subsystem1/MPTA_Process/Variant Subsystem ==
  note: 1) Add Subsystem or Model blocks as valid variant choices.
      | 2) You cannot connect blocks at this level. At simulation, connectivity is automatically
      | determined, based on the active variant and port name matching.
  Te* : Inport
  (Ld-Lq)^2 : Inport  Port=2
  Direct calculation : Subsystem  VariantControl=MPTA_Way==0
  Leading angle : Subsystem  VariantControl=MPTA_Way==1
  Iq : Outport

== system backbone/Variant Subsystem/MPTA_MPTV_PMSM/MPTA_弱磁/MPTA_MPTV_Base_Te/Variant Subsystem/PID ==
  In1 : Inport
  Speed : Subsystem  AncestorBlock=|  DialogController=POWERSYS.PowerSysDialog  mask(Discrete PI Controller){Kpw=0.14, Kiw=0.14*50, Ba=0, Par_Limits=[800 -800], Init=0, Ts=Ts}
      | powerlib_extras/Discrete 
      | Control Blocks/Discrete
      | PI Controller
      mask prompts: Kpw "Proportional gain (Kp):"; Kiw "Integral gain (Ki):"; Ba "feedback gain (Ba)"; Par_Limits "Output limits: [ Upper   Lower ]"; Init "Output initial value:"; Ts "Sample time:"
      mask help: This block implements a discrete PI controller.
      mask init:
      | UpperLimit=Par_Limits(1);
      | LowerLimit=Par_Limits(2);
      | power_initmask();
      settings: LibrarySourceBlock=|
      | powerlib_extras/Discrete
      | Control Blocks/Discrete
      | PI Controller
      mask Help: This block is part of a subset of blocks in the Extras library that does not have documentation associated with it, other than the block mask description.
      mask Display: disp('PI');
  Speed1 : Subsystem  Commented=on  AncestorBlock=|  DialogController=POWERSYS.PowerSysDialog  mask(Discrete PI Controller){Kpw=0.14, Kiw=0.14*50, Ba=0, Par_Limits=[800 -800], Init=0, Ts=Ts}
      | powerlib_extras/Discrete 
      | Control Blocks/Discrete
      | PI Controller
      mask prompts: Kpw "Proportional gain (Kp):"; Kiw "Integral gain (Ki):"; Ba "feedback gain (Ba)"; Par_Limits "Output limits: [ Upper   Lower ]"; Init "Output initial value:"; Ts "Sample time:"
      mask help: This block implements a discrete PI controller.
      mask init:
      | UpperLimit=Par_Limits(1);
      | LowerLimit=Par_Limits(2);
      | power_initmask();
      settings: LibrarySourceBlock=|
      | powerlib_extras/Discrete
      | Control Blocks/Discrete
      | PI Controller
      mask Help: This block is part of a subset of blocks in the Extras library that does not have documentation associated with it, other than the block mask description.
      mask Display: disp('PI');
  Te* : Outport
  wires:
  Speed/1(Out) -> Te*/1
  In1/1 -> Speed/1(Error)

== system backbone/Variant Subsystem/MPTA_MPTV_PMSM/MPTA_弱磁/MPTA_MPTV_Base_Te/Variant Subsystem/SMC ==
  In1 : Inport
  Speed4 : Subsystem  AncestorBlock=|  DialogController=POWERSYS.PowerSysDialog  mask(Discrete PI Controller){C=60, Mu=200, q=300, Par_Limits=[1000 -1000], Init=0, Ts=0.000001}
      | powerlib_extras/Discrete 
      | Control Blocks/Discrete
      | PI Controller
      mask prompts: C "Gain (c):"; Mu "Gain (Mu):"; q "Gain (q)"; Par_Limits "Output limits: [ Upper   Lower ]"; Init "Output initial value:"; Ts "Sample time:"
      mask help: This block implements a discrete PI controller.
      mask init:
      | UpperLimit=Par_Limits(1);
      | LowerLimit=Par_Limits(2);
      | power_initmask();
      settings: LibrarySourceBlock=|
      | powerlib_extras/Discrete
      | Control Blocks/Discrete
      | PI Controller
      mask Help: This block is part of a subset of blocks in the Extras library that does not have documentation associated with it, other than the block mask description.
      mask Display: disp('SMC');
  Te* : Outport
  wires:
  Speed4/1(Out) -> Te*/1
  In1/1 -> Speed4/1(Error)

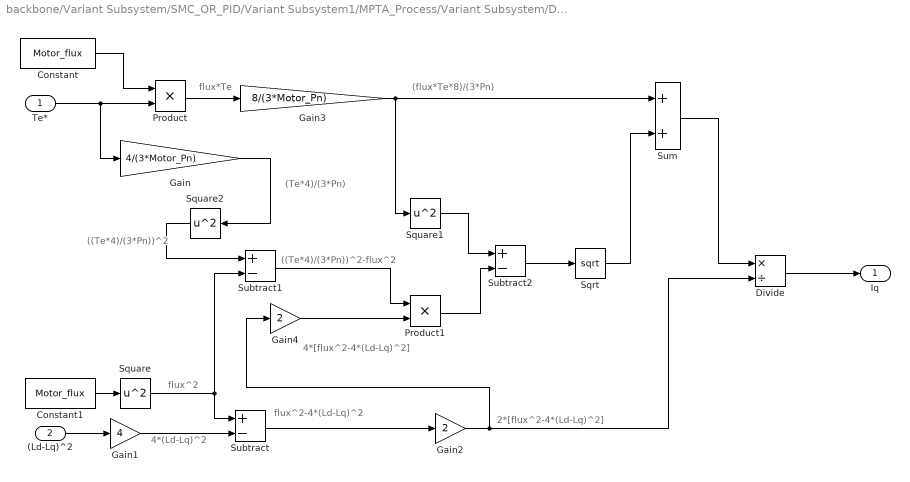
== system backbone/Variant Subsystem/SMC_OR_PID/Variant Subsystem1/MPTA_Process/Variant Subsystem/Direct calculation ==
  note: 4*[flux^2-4*(Ld-Lq)^2]
  note: 2*[flux^2-4*(Ld-Lq)^2]
  note: flux^2-4*(Ld-Lq)^2
  note: 4*(Ld-Lq)^2
  note: ((Te*4)/(3*Pn))^2-flux^2
  note: flux^2
  note: ((Te*4)/(3*Pn))^2
  note: (Te*4)/(3*Pn)
  note: (flux*Te*8)/(3*Pn)
  note: flux*Te
  Te* : Inport
  (Ld-Lq)^2 : Inport  Port=2
  Constant : Constant  Value=Motor_flux
  Constant1 : Constant  Value=Motor_flux
  Divide : Product  Inputs=*/
  Gain : Gain  Gain=4/(3*Motor_Pn)
  Gain1 : Gain  Gain=4
  Gain2 : Gain  Gain=2
  Gain3 : Gain  Gain=8/(3*Motor_Pn)
  Gain4 : Gain  Gain=2
  Product : Product
  Product1 : Product
  Sqrt : Sqrt
  Square : Math  Operator=square
  Square1 : Math  Operator=square
  Square2 : Math  Operator=square
  Subtract : Sum  Inputs=+-
  Subtract1 : Sum  Inputs=+-
  Subtract2 : Sum  Inputs=+-
  Sum : Sum
  Iq : Outport
  wires:
  Te*/1 -> Product/2, Gain/1
  Constant/1 -> Product/1
  Constant1/1 -> Square/1
  (Ld-Lq)^2/1 -> Gain1/1
  Subtract/1 -> Gain2/1
  Product/1 -> Gain3/1
  Gain3/1 -> Square1/1, Sum/1
  Gain1/1 -> Subtract/2
  Square/1 -> Subtract/1, Subtract1/2
  Gain2/1 -> Divide/2, Gain4/1
  Gain4/1 -> Product1/2
  Subtract1/1 -> Product1/1
  Square1/1 -> Subtract2/1
  Product1/1 -> Subtract2/2
  Subtract2/1 -> Sqrt/1
  Sqrt/1 -> Sum/2
  Sum/1 -> Divide/1
  Divide/1 -> Iq/1
  Gain/1 -> Square2/1
  Square2/1 -> Subtract1/1

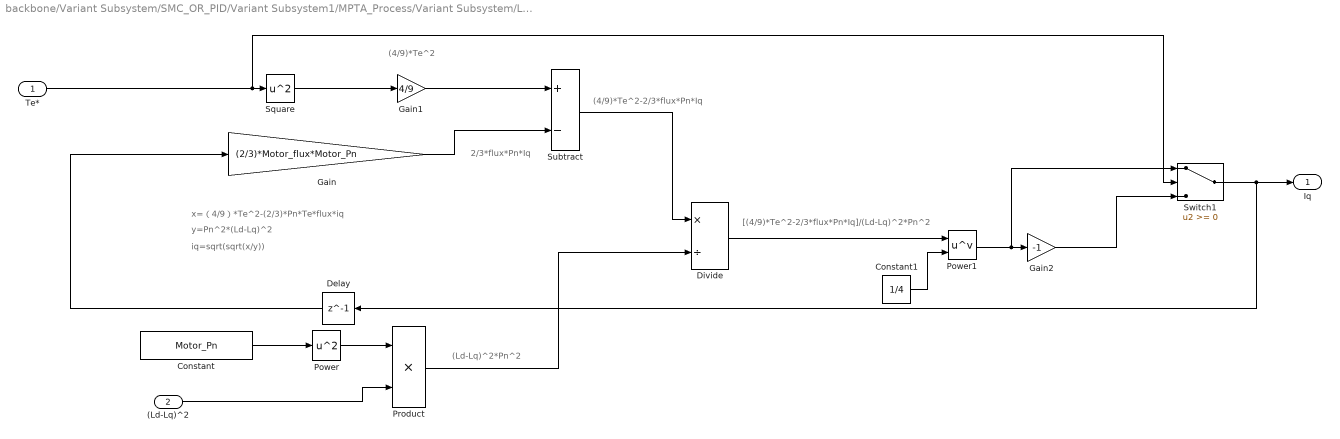
== system backbone/Variant Subsystem/SMC_OR_PID/Variant Subsystem1/MPTA_Process/Variant Subsystem/Leading angle ==
  note: [(4/9)*Te^2-2/3*flux*Pn*Iq]/(Ld-Lq)^2*Pn^2
  note: (4/9)*Te^2-2/3*flux*Pn*Iq
  note: (4/9)*Te^2
  note: 2/3*flux*Pn*Iq
  note: (Ld-Lq)^2*Pn^2
  note: iq=sqrt(sqrt(x/y))
  note: y=Pn^2*(Ld-Lq)^2
  note: x=（4/9）*Te^2-(2/3)*Pn*Te*flux*iq
  Te* : Inport
  (Ld-Lq)^2 : Inport  Port=2
  Constant : Constant  Value=Motor_Pn
  Constant1 : Constant  Value=1/4
  Delay : Delay  DelayLength=1  InitialCondition=0  SampleTime=0.000001
  Divide : Product  Inputs=*/
  Gain : Gain  Gain=(2/3)*Motor_flux*Motor_Pn
  Gain1 : Gain  Gain=4/9
  Gain2 : Gain  Gain=-1
  Power : Math  Operator=square
  Power1 : Math  Operator=pow
  Product : Product
  Square : Math  Operator=square
  Subtract : Sum  Inputs=+-
  Switch1 : Switch  SaturateOnIntegerOverflow=off  InputSameDT=off
  Iq : Outport
  wires:
  Constant/1 -> Power/1
  Power/1 -> Product/1
  (Ld-Lq)^2/1 -> Product/2
  Te*/1 -> Switch1/2, Square/1
  Square/1 -> Gain1/1
  Subtract/1 -> Divide/1
  Product/1 -> Divide/2
  Divide/1 -> Power1/1
  Gain1/1 -> Subtract/1
  Gain/1 -> Subtract/2
  Constant1/1 -> Power1/2
  Delay/1 -> Gain/1
  ? -> ?
  Power1/1 -> Switch1/1, Gain2/1
  Gain2/1 -> Switch1/3
  Switch1/1 -> Delay/1, Iq/1

== system backbone/Variant Subsystem/MPTA_MPTV_PMSM/MPTA_弱磁/MPTA_MPTV_Base_Te/Variant Subsystem/PID/Speed ==
  note: Pierre Giroux, Gilbert Sybille
      | Power System Simulation Laboratory
      | IREQ, Hydro-Quebc
  note: Discrete PID Controller
  Error : Inport  SampleTime=Ts
  Discrete-Time Integrator : DiscreteIntegrator  InitialCondition=Init  SampleTime=Ts  LimitOutput=on  UpperSaturationLimit=UpperLimit  LowerSaturationLimit=LowerLimit  ICPrevOutput=DiscIntNeverNeededParam  ICPrevScaledInput=DiscIntNeverNeededParam
  Kp1 : Gain  Gain=Ba  SaturateOnIntegerOverflow=on  SampleTime=Ts  OutDataTypeStr=Inherit: Same as input  ParamDataTypeStr=Inherit: Same as input
  Kp4 : Gain  Gain=Kpw  SaturateOnIntegerOverflow=on  SampleTime=Ts  OutDataTypeStr=Inherit: Same as input  ParamDataTypeStr=Inherit: Same as input
  Kp5 : Gain  Gain=Kiw  SaturateOnIntegerOverflow=on  SampleTime=Ts  OutDataTypeStr=Inherit: Same as input  ParamDataTypeStr=Inherit: Same as input
  Saturation2 : Saturate  UpperLimit=UpperLimit  LowerLimit=LowerLimit  SampleTime=Ts
  Sum6 : Sum  Inputs=++-  InputSameDT=on  SaturateOnIntegerOverflow=on  SampleTime=Ts  OutDataTypeStr=Inherit: Same as first input
  Zero-Order Hold : ZeroOrderHold  SampleTime=Ts
  Out : Outport  SampleTime=Ts  InitialOutput=0
  wires:
  Kp1/1 -> Sum6/3
  Sum6/1 -> Saturation2/1
  Kp5/1 -> Discrete-Time Integrator/1
  Kp4/1 -> Zero-Order Hold/1
  Discrete-Time Integrator/1 -> Sum6/2
  Saturation2/1 -> Out/1
  Zero-Order Hold/1 -> Sum6/1
  Error/1 -> Kp4/1, Kp5/1, Kp1/1

== system backbone/Variant Subsystem/MPTA_MPTV_PMSM/MPTA_弱磁/MPTA_MPTV_Base_Te/Variant Subsystem/PID/Speed1 ==
  note: Discrete PID Controller
  note: Pierre Giroux, Gilbert Sybille
      | Power System Simulation Laboratory
      | IREQ, Hydro-Quebc
  Error : Inport  SampleTime=Ts
  Discrete-Time Integrator : DiscreteIntegrator  InitialCondition=Init  SampleTime=Ts  LimitOutput=on  UpperSaturationLimit=UpperLimit  LowerSaturationLimit=LowerLimit  ICPrevOutput=DiscIntNeverNeededParam  ICPrevScaledInput=DiscIntNeverNeededParam
  Kp1 : Gain  Gain=Ba  SaturateOnIntegerOverflow=on  SampleTime=Ts  OutDataTypeStr=Inherit: Same as input  ParamDataTypeStr=Inherit: Same as input
  Kp4 : Gain  Gain=Kpw  SaturateOnIntegerOverflow=on  SampleTime=Ts  OutDataTypeStr=Inherit: Same as input  ParamDataTypeStr=Inherit: Same as input
  Kp5 : Gain  Gain=Kiw  SaturateOnIntegerOverflow=on  SampleTime=Ts  OutDataTypeStr=Inherit: Same as input  ParamDataTypeStr=Inherit: Same as input
  Saturation2 : Saturate  UpperLimit=UpperLimit  LowerLimit=LowerLimit  SampleTime=Ts
  Sum6 : Sum  Inputs=++-  InputSameDT=on  SaturateOnIntegerOverflow=on  SampleTime=Ts  OutDataTypeStr=Inherit: Same as first input
  Zero-Order Hold : ZeroOrderHold  SampleTime=Ts
  Out : Outport  SampleTime=Ts  InitialOutput=0
  wires:
  Error/1 -> Kp1/1, Kp5/1, Kp4/1
  Zero-Order Hold/1 -> Sum6/1
  Saturation2/1 -> Out/1
  Discrete-Time Integrator/1 -> Sum6/2
  Kp4/1 -> Zero-Order Hold/1
  Kp5/1 -> Discrete-Time Integrator/1
  Sum6/1 -> Saturation2/1
  Kp1/1 -> Sum6/3

== system backbone/Variant Subsystem/MPTA_MPTV_PMSM/MPTA_弱磁/MPTA_MPTV_Base_Te/Variant Subsystem/SMC/Speed4 ==
  Error : Inport  SampleTime=Ts
  1/D : Gain  Gain=1/(1.5*Pn*flux/0.003)  SaturateOnIntegerOverflow=on  SampleTime=Ts  OutDataTypeStr=Inherit: Same as input  ParamDataTypeStr=Inherit: Same as input
  Discrete Derivative : simulink/Discrete/Discrete Derivative  gainval=1.0  ICPrevScaledInput=0.0  OutMin=[]  OutMax=[]  OutDataType=fixdt(1, 16)  OutScaling=2^-10  DoSatur=off
  Discrete-Time Integrator : DiscreteIntegrator  InitialCondition=0.001  SampleTime=Ts  ICPrevOutput=DiscIntNeverNeededParam  ICPrevScaledInput=DiscIntNeverNeededParam
  Kp1 : Gain  Gain=q  SaturateOnIntegerOverflow=on  SampleTime=Ts  OutDataTypeStr=Inherit: Same as input  ParamDataTypeStr=Inherit: Same as input
  Kp2 : Gain  Gain=Mu  SaturateOnIntegerOverflow=on  SampleTime=Ts  OutDataTypeStr=Inherit: Same as input  ParamDataTypeStr=Inherit: Same as input
  Kp3 : Gain  Gain=C  SaturateOnIntegerOverflow=on  SampleTime=Ts  OutDataTypeStr=Inherit: Same as input  ParamDataTypeStr=Inherit: Same as input
  Kp4 : Gain  Gain=C  SaturateOnIntegerOverflow=on  SampleTime=Ts  OutDataTypeStr=Inherit: Same as input  ParamDataTypeStr=Inherit: Same as input
  Nr->wm : Gain  Gain=pi/30  SaturateOnIntegerOverflow=on  SampleTime=Ts  OutDataTypeStr=Inherit: Same as input  ParamDataTypeStr=Inherit: Same as input
  Saturation2 : Saturate  UpperLimit=UpperLimit  LowerLimit=LowerLimit  SampleTime=Ts
  Sign : Signum
  Sum1 : Sum  InputSameDT=on  SaturateOnIntegerOverflow=on  SampleTime=Ts  OutDataTypeStr=Inherit: Same as first input
  Sum2 : Sum  Inputs=++-  InputSameDT=on  SaturateOnIntegerOverflow=on  SampleTime=Ts  OutDataTypeStr=Inherit: Same as first input
  Out : Outport  SampleTime=Ts  InitialOutput=0
  wires:
  Nr->wm/1 -> Kp4/1, Discrete Derivative/1
  Discrete-Time Integrator/1 -> 1/D/1
  1/D/1 -> Saturation2/1
  Kp3/1 -> Sum2/3
  Kp2/1 -> Sum2/2
  Sum1/1 -> Kp1/1, Sign/1
  Sign/1 -> Kp2/1
  Kp1/1 -> Sum2/1
  Error/1 -> Nr->wm/1
  Sum2/1 -> Discrete-Time Integrator/1
  Discrete Derivative/1 -> Sum1/2, Kp3/1
  Saturation2/1 -> Out/1
  Kp4/1 -> Sum1/1

== matlab function backbone/MATLAB Function ==
  data: SysCtrlWay input; u input; y output
function y = fcn(SysCtrlWay, u)

if SysCtrlWay==5 % 当弱磁控制时采用这个时间变换
    if u<0.2
        y=2000;
    elseif u>0.2&&u<0.5
        y=3000;
    elseif u>0.5&&u<0.8
        y=6000;
    elseif u>0.8
        y=1000;    
    else
        y=1000; 
    end
else
    y=2000;
end
end

== matlab function backbone/Variant Subsystem/DTC_PMSM/定子磁链和电磁转矩估计/电压法估计磁链/sector ==
  data: fluxalpha input; fluxbeta input; N output
function N = fcn(fluxalpha,fluxbeta)

if(fluxalpha==0) 
    N=1;    %如果输入值为0，电压参考量在第一扇区
else
    a1=fluxalpha; 
    b1=fluxalpha*(-0.5)+sqrt(3)*fluxbeta; %%根据文章的计算公式得到
    c1=fluxalpha*(-0.5)-(sqrt(3)/2)*fluxbeta;
    if a1>0
        a=0;
    else
        a=1;
    end
    if b1>0
        b=0;
    else
        b=1;
    end
    if c1>0
        c=0;
    else
        c=1;
    end
    N1=4*a+2*b+c; %扇区计算
    Sector_table=[2 6 1 4 3 5];
    N=Sector_table(N1);
end

== matlab function backbone/Variant Subsystem/SMC_OR_PID/Variant Subsystem2/EKF_αβ/MATLAB Function ==
  data: ialpha input; theta output; ibeta input; ualpha input; ubeta input; Ts input; Ls input; Rs input; flux input; we output

function [theta, we] = EKF(ialpha, ibeta, ualpha, ubeta, Ts, Ls, Rs, flux)

% 声明持久变量
persistent x_k_1 P_K_1

% 如果持久变量为空，则进行初始化
if isempty(x_k_1)
    x_k_1 = double([0, 0, 0, 0]');
end   
if isempty(P_K_1)
    P_K_1 = double(diag([0.1, 0.1, 0, 0]));
end 

% 输入向量
Is = double([ialpha ibeta]');
Us = double([ualpha ubeta]');

% 系统噪声和测量噪声协方差矩阵
Q = double(diag([0.1 0.1 1 0.01]));
R = double(diag([0.2 0.2]));

% 系统矩阵和控制矩阵
C = double([1 0 0 0;0 1 0 0]);
B = double([1/Ls 0;0 1/Ls;0 0;0 0]);

% 状态方程和状态转移矩阵
f = double([-Rs*x_k_1(1,1)/Ls + x_k_1(3,1)*flux*sin(x_k_1(4,1))/Ls;
            -Rs*x_k_1(2,1)/Ls - x_k_1(3,1)*flux*cos(x_k_1(4,1))/Ls;
            0;
            x_k_1(3,1)]);
F = double([-Rs/Ls 0 flux*sin(x_k_1(4,1))/Ls flux*x_k_1(3,1)*cos(x_k_1(4,1))/Ls;
            0 -Rs/Ls -flux*cos(x_k_1(4,1))/Ls flux*x_k_1(3,1)*sin(x_k_1(4,1))/Ls;
            0 0 0 0;
            0 0 1 0]);

%v=diag([1,1,1,1])+Ts*F;
% 计算预测值
X_pred = x_k_1 + Ts * (f + B * Us);
Y_Pred = C * X_pred;
Y = Is;

% 计算预测误差协方差
P_Pred = P_K_1 + Ts * (F * P_K_1 + P_K_1 * F') + Q;
%P_Pred=v*P_K_1*v'+Q;

% 计算卡尔曼增益
K = P_Pred * C' * inv(C * P_Pred * C' + R);

% 修正预测值
x_hat = X_pred + K * (Y - Y_Pred);

% 更新误差协方差
P_hat = P_Pred - K * C * P_Pred;

% 输出更新后的状态值
we = double(x_hat(3,1));
theta = double(x_hat(4,1));

% 更新持久变量
x_k_1=x_hat;
P_K_1 = P_hat;

end

== matlab function backbone/Variant Subsystem/DTC_PMSM/PWM/PMSM_switch ==
  data: Flux input; Torque input; Table output; N input
function Table = fcn(Flux, Torque, N)
 %%根据文章的表格计算得到
%V_Table=[2 4 6 1 3 5;4 1 5 2 6 3;3 6 2 5 1 4 ;5 3 1 6 4 2];
%[1,1,1,0,0,0] [1,0,0,1,1,0] [0,1,0,1,0,1]


%https://blog.csdn.net/m0_70748084/article/details/126374001
V_Table=[5 6 1 2 3 4;3 4 5 6 1 2;6 1 2 3 4 5;2 3 4 5 6 1];
%[1,1,0,0,0,1] [0,1,1,1,0,0] [0,0,0,1,1,1]
x=2*Flux+Torque+1;
Table=V_Table(x,N);
